simulink model "robot_soccer_sim"  (R2015b)
settings: Solver=ode45  StartTime=0.0  StopTime=60  RelTol=1e-3
InitFcn:
  | param
undefined symbols (not defined in the file or in its folder): controller_home, controller_walle, drawEnvironment, lowlevelctrl, P, robot_change_frames
settings Model: Creator=beard  LastModifiedBy=mach
settings DataIOCC: SaveFormat=Array
settings DebuggingCC: UnderspecifiedInitializationDetection=Classic  MergeDetectMultiDrivingBlocksExec=none  SolverPrmCheckMsg=warning  StateNameClashWarn=warning
settings HardwareCC: ProdBitPerPointer=32  ProdLargestAtomicFloat=None  ProdIntDivRoundTo=Undefined  ProdEndianess=Unspecified  ProdWordSize=32  ProdHWDeviceType=32-bit Generic
settings GRTTargetCC: GeneratePreprocessorConditionals=Disable all
settings ConfigComp: CovModelRefEnable=Off  CovSFcnEnable=off

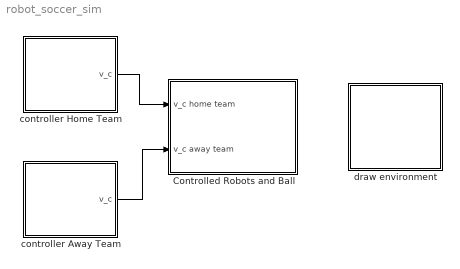
== system robot_soccer_sim ==
  "Controlled Robots and Ball " : Subsystem
      mask Display: image(imread('cmu_2002_diffbot.jpg'))
  controller Away Team : Subsystem
      mask Display: image(imread('minnowboard.png'))
  controller Home Team : Subsystem
      mask Display: image(imread('minnowboard.png'))
  draw environment : Subsystem
      mask Display: image(imread('ssl_game.jpg'))
  wires:
  controller Away Team/1(v_c) -> "Controlled Robots and Ball "/2(v_c away team)
  controller Home Team/1(v_c) -> "Controlled Robots and Ball "/1(v_c home team)

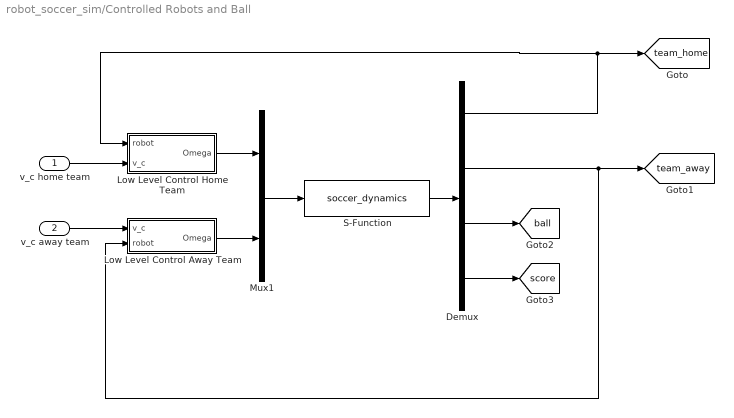
== system robot_soccer_sim/Controlled Robots and Ball  ==
  v_c home team : Inport
  v_c away team : Inport  Port=2
  Demux : Demux  Outputs=[3*P.num_robots; 3*P.num_robots; 2; 2]
  Low Level Control Home Team : Subsystem
  Low Level Control Away Team : Subsystem
  Mux1 : Mux  Inputs=2
  S-Function : S-Function  FunctionName=soccer_dynamics  Parameters=P  SFunctionDeploymentMode=off  EnableBusSupport=off
  tag scope: ball=global, score=global, team_away=global, team_home=global
  wires:
  Mux1/1 -> S-Function/1
  Demux/3 -> [ball]
  S-Function/1 -> Demux/1
  Demux/1 -> Low Level Control Home Team/1(robot), [team_home]
  Low Level Control Home Team/1(Omega) -> Mux1/1
  Low Level Control Away Team/1(Omega) -> Mux1/2
  Demux/2 -> Low Level Control Away Team/2(robot), [team_away]
  v_c home team/1 -> Low Level Control Home Team/2(v_c)
  v_c away team/1 -> Low Level Control Away Team/1(v_c)
  Demux/4 -> [score]

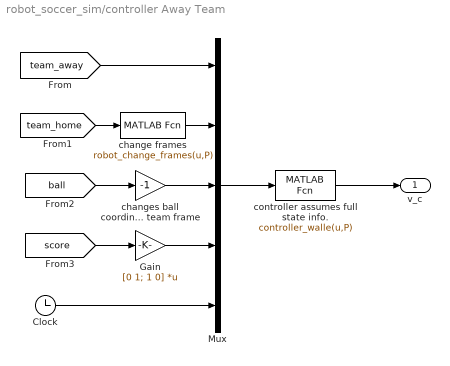
== system robot_soccer_sim/controller Away Team ==
  Clock : Clock
  Gain : Gain  Gain=[0 1; 1 0]  Multiplication=Matrix(K*u)
  Mux : Mux  Inputs=5
  "change frames " : MATLABFcn  MATLABFcn=robot_change_frames(u,P)  OutputDimensions=3*P.num_robots  SampleTime=P.control_sample_rate
  changes ball coordinates to away team frame : Gain  Gain=-1
  controller assumes full state info. : MATLABFcn  MATLABFcn=controller_walle(u,P)  OutputDimensions=3*P.num_robots  SampleTime=P.control_sample_rate
  v_c : Outport
  wires:
  Mux/1 -> controller assumes full state info./1
  [team_away] -> Mux/1
  Clock/1 -> Mux/5
  "change frames "/1 -> Mux/2
  [team_home] -> "change frames "/1
  [ball] -> changes ball coordinates to away team frame/1
  changes ball coordinates to away team frame/1 -> Mux/3
  [score] -> Gain/1
  Gain/1 -> Mux/4
  controller assumes full state info./1 -> v_c/1

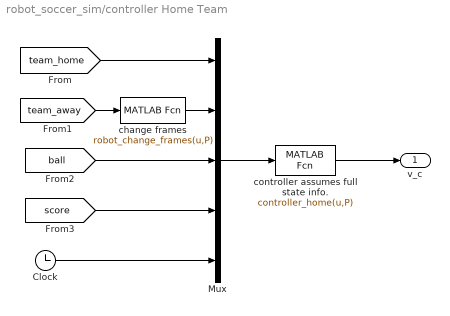
== system robot_soccer_sim/controller Home Team ==
  Clock : Clock
  Mux : Mux  Inputs=5
  "change frames " : MATLABFcn  MATLABFcn=robot_change_frames(u,P)  OutputDimensions=3*P.num_robots  SampleTime=P.control_sample_rate
  controller assumes full state info. : MATLABFcn  MATLABFcn=controller_home(u,P)  OutputDimensions=3*P.num_robots  SampleTime=P.control_sample_rate
  v_c : Outport
  wires:
  Mux/1 -> controller assumes full state info./1
  [team_home] -> Mux/1
  [ball] -> Mux/3
  Clock/1 -> Mux/5
  controller assumes full state info./1 -> v_c/1
  "change frames "/1 -> Mux/2
  [team_away] -> "change frames "/1
  [score] -> Mux/4

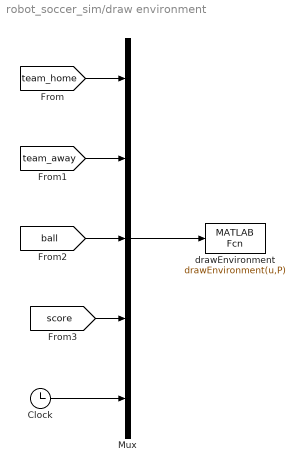
== system robot_soccer_sim/draw environment ==
  Clock : Clock
  Mux : Mux  Inputs=5
  drawEnvironment : MATLABFcn  MATLABFcn=drawEnvironment(u,P)  OutputDimensions=0  SampleTime=P.display_rate
  wires:
  Mux/1 -> drawEnvironment/1
  [team_home] -> Mux/1
  [team_away] -> Mux/2
  [ball] -> Mux/3
  [score] -> Mux/4
  Clock/1 -> Mux/5

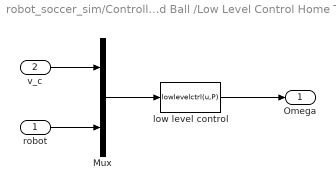
== system robot_soccer_sim/Controlled Robots and Ball /Low Level Control Home Team ==
  robot : Inport
  v_c : Inport  Port=2
  Mux : Mux  Inputs=2
  low level control : MATLABFcn  MATLABFcn=lowlevelctrl(u,P)  OutputDimensions=3*P.num_robots  SampleTime=0.01
  Omega : Outport
  wires:
  v_c/1 -> Mux/1
  robot/1 -> Mux/2
  Mux/1 -> low level control/1
  low level control/1 -> Omega/1

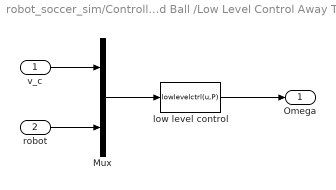
== system robot_soccer_sim/Controlled Robots and Ball /Low Level Control Away Team ==
  v_c : Inport
  robot : Inport  Port=2
  Mux : Mux  Inputs=2
  low level control : MATLABFcn  MATLABFcn=lowlevelctrl(u,P)  OutputDimensions=3*P.num_robots  SampleTime=0.01
  Omega : Outport
  wires:
  v_c/1 -> Mux/1
  robot/1 -> Mux/2
  Mux/1 -> low level control/1
  low level control/1 -> Omega/1
